simulink model "discontinuidades"  (R2021a)
settings: Solver=VariableStepAuto  StartTime=0.0  StopTime=10.0  MaxStep=0.01  RelTol=1e-3
libraries: simulink x1
settings Model: Creator=Aula  LastModifiedBy=Aula

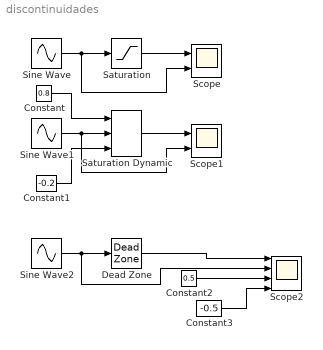
== system discontinuidades ==
  Constant : Constant  Value=0.8
  Constant1 : Constant  Value=-0.2
  Constant2 : Constant  Value=0.5
  Constant3 : Constant  Value=-0.5
  Dead Zone : DeadZone  SaturateOnIntegerOverflow=on
  Saturation : Saturate
  Saturation Dynamic : simulink/Discontinuities/Saturation Dynamic  OutMin=[]  OutMax=[]  OutDataTypeStr=Inherit: Same as second input  OutDataType=fixdt(1, 16)  OutScaling=2^-10  DoSatur=off
  Scope : Scope  NumInputPorts=2
  Scope1 : Scope  NumInputPorts=2
  Scope2 : Scope  NumInputPorts=4
  Sine Wave : Sin  SampleTime=0
  Sine Wave1 : Sin  SampleTime=0
  Sine Wave2 : Sin  SampleTime=0
  wires:
  Sine Wave/1 -> Scope/2, Saturation/1
  Saturation/1 -> Scope/1
  Saturation Dynamic/1 -> Scope1/1
  Sine Wave1/1 -> Saturation Dynamic/2, Scope1/2
  Constant/1 -> Saturation Dynamic/1
  Constant1/1 -> Saturation Dynamic/3
  Dead Zone/1 -> Scope2/1
  Sine Wave2/1 -> Dead Zone/1, Scope2/2
  Constant2/1 -> Scope2/3
  Constant3/1 -> Scope2/4
